simulink model "fz7_2"  (R2014a)
settings: Solver=ode45  StartTime=0.0  StopTime=50000  RelTol=1e-3
values from neighbouring files (symbols this model uses):
  SymbolRate = 1000    [eg7_11.m]    (also in eg7_2.m = 2; eg7_4.m = 2; eg7_7.m = 2)
libraries: commutil2 x4, commsink2 x2, commdigbbndam3 x2, commchan3 x1, commfilt2 x1, commrandsrc2 x1
settings Model: Creator=tzb  LastModifiedBy=tzb
settings DebuggingCC: SolverPrmCheckMsg=none

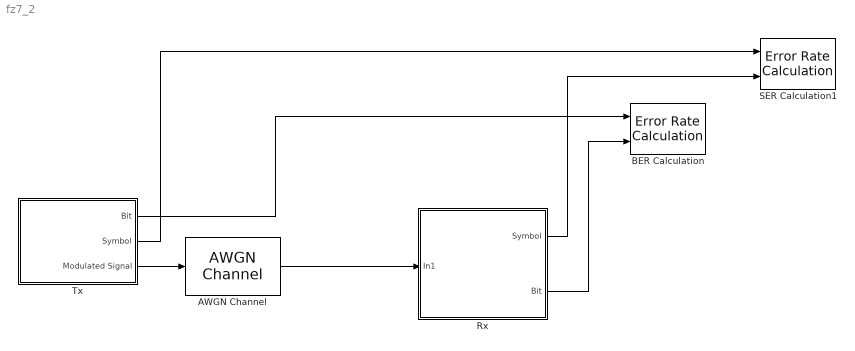
== system fz7_2 ==
  AWGN Channel : commchan3/AWGN Channel  InputProcessing=Columns as channels (frame based)  seed=67  noiseMode="Signal to noise ratio  (Es/No)"  EbNodB=SNR  EsNodB=SNR  SNRdB=10  bitsPerSym=1  Ps=5  Tsym=1/SymbolRate  variance=1
  BER Calculation : commsink2/Error Rate Calculation  N=0  st_delay=SymbolRate*2  cp_mode=Entire frame  subframe=[]  PMode=Workspace  WsName=BER  RsMode2=off  stop=off  numErr=100  maxBits=1e6
  Rx : Subsystem
  SER Calculation1 : commsink2/Error Rate Calculation  N=0  st_delay=SymbolRate  cp_mode=Entire frame  subframe=[]  PMode=Workspace  WsName=SER  RsMode2=off  stop=off  numErr=100  maxBits=1e6
  Tx : Subsystem
  wires:
  Tx/3(Modulated Signal) -> AWGN Channel/1
  AWGN Channel/1 -> Rx/1(In1)
  Rx/2(Bit) -> BER Calculation/2
  Tx/1(Bit) -> BER Calculation/1
  Rx/1("Symbol ") -> SER Calculation1/2
  Tx/2(Symbol) -> SER Calculation1/1

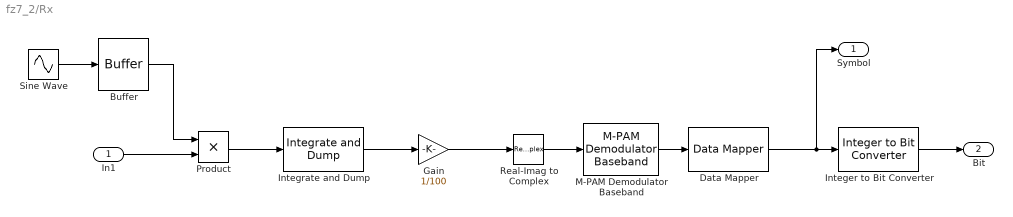
== system fz7_2/Rx ==
  In1 : Inport
  Buffer : Buffer  N=100*SymbolRate
  Data Mapper : commutil2/Data Mapper  MapMode=Gray to Binary  M=4  MapVec=[0 1 3 2 7 6 4 5]
  Gain : Gain  Gain=1/100
  Integer to Bit Converter : commutil2/Integer to Bit Converter  nbits=2  signedInputValues=Unsigned  bitOrder=MSB first  outDtype=Inherit via internal rule
  Integrate and Dump : commfilt2/Integrate and Dump  obssamples=100  offsetsamples=0  nodump=off  roundingMode=Floor  overflowMode=off
  M-PAM Demodulator Baseband : commdigbbndam3/M-PAM Demodulator Baseband  M=4  OutType=Integer  Dec=Gray  PowType=Min. distance between symbols  MinDist=2  AvgPow=1  PeakPow=1  outDtype1=Inherit via internal rule  outDtype2=Inherit via internal rule  denormFactorWordLen=16  prodOutWordLen=16  prodOutRoundingMode=Floor  prodOutOverflowMode=Wrap  sumWordLen=16
  Product : Product  RndMeth=Zero
  Real-Imag to Complex : RealImagToComplex  Input=Real
  Sine Wave : Sin  Amplitude=sqrt(2)  Frequency=2*pi*SymbolRate  Phase=pi/2  SampleTime=1/(100*SymbolRate)
  "Symbol " : Outport
  Bit : Outport  Port=2
  wires:
  Integrate and Dump/1 -> Gain/1
  Integer to Bit Converter/1 -> Bit/1
  Product/1 -> Integrate and Dump/1
  Real-Imag to Complex/1 -> M-PAM Demodulator Baseband/1
  Data Mapper/1 -> "Symbol "/1, Integer to Bit Converter/1
  Gain/1 -> Real-Imag to Complex/1
  M-PAM Demodulator Baseband/1 -> Data Mapper/1
  Sine Wave/1 -> Buffer/1
  In1/1 -> Product/2
  Buffer/1 -> Product/1

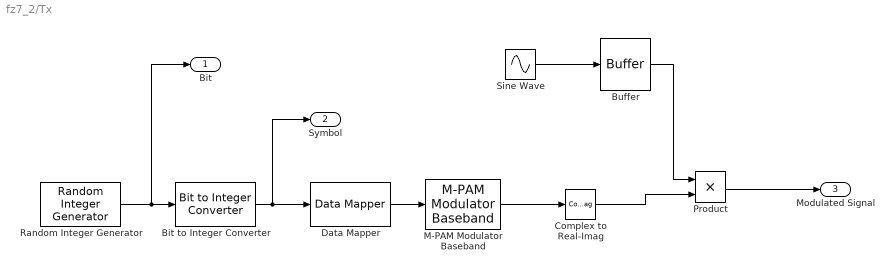
== system fz7_2/Tx ==
  Bit to Integer Converter : commutil2/Bit to Integer Converter  nbits=2  bitOrder=MSB first  signedOutputValues=Unsigned  outDtype=Same as input  outDtypeSigned=Inherit via internal rule
  Buffer : Buffer  N=100*SymbolRate
  Complex to Real-Imag : ComplexToRealImag  Output=Real
  Data Mapper : commutil2/Data Mapper  MapMode=Binary to Gray  M=4  MapVec=[0 1 3 2 7 6 4 5]
  M-PAM Modulator Baseband : commdigbbndam3/M-PAM Modulator Baseband  M=4  InType=Integer  Enc=Gray  PowType=Min. distance between symbols  MinDist=2  AvgPow=1  PeakPow=1  outDtype=double  outWordLen=16  outUDDataType=sfix(16)  outFracLenMode=Best precision  outFracLen=15
  Product : Product  RndMeth=Zero
  Random Integer Generator : commrandsrc2/Random Integer Generator  mul=2  seed=37  Ts=1/(2*SymbolRate)  frameBased=on  sampPerFrame=2*SymbolRate  orient=off  outDataType=double
  Sine Wave : Sin  Amplitude=sqrt(2)  Frequency=2*pi*SymbolRate  Phase=pi/2  SampleTime=1/(100*SymbolRate)
  Bit : Outport
  Symbol : Outport  Port=2
  Modulated Signal : Outport  Port=3
  wires:
  M-PAM Modulator Baseband/1 -> Complex to Real-Imag/1
  Random Integer Generator/1 -> Bit/1, Bit to Integer Converter/1
  Product/1 -> Modulated Signal/1
  Sine Wave/1 -> Buffer/1
  Complex to Real-Imag/1 -> Product/2
  Bit to Integer Converter/1 -> Symbol/1, Data Mapper/1
  Data Mapper/1 -> M-PAM Modulator Baseband/1
  Buffer/1 -> Product/1
